simulink model "AMCLIB_FW_BAM_F32"  (Simulink 8.3)
settings: Solver=ode45  StartTime=0.0  StopTime=10.0  RelTol=1e-3
undefined symbols (not defined in the file): f32IntegGainFW, f32PropGainFW, s16IntegGainShiftFW, s16PropGainShiftFW, u16NSamplesFW
settings Model: Creator=B37097  LastModifiedBy=B37097
settings DataIOCC: SignalLoggingSaveFormat=Dataset
settings DebuggingCC: UnderspecifiedInitializationDetection=Simplified  StateNameClashWarn=none
settings GRTTargetCC: CombineOutputUpdateFcns=on  GRTInterface=off

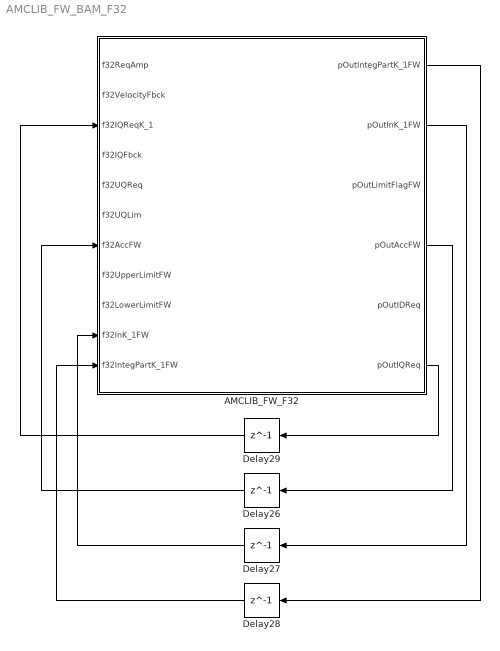
== system AMCLIB_FW_BAM_F32 ==
  AMCLIB_FW_F32 : Subsystem  mask(AMCLIB_FW_F32){u16NSamplesFW=u16NSamplesFW, f32PropGainFW=f32PropGainFW, s16PropGainShiftFW=s16PropGainShiftFW, f32IntegGainFW=f32IntegGainFW, s16IntegGainShiftFW=s16IntegGainShiftFW}
      mask help: Bit accurate model of the speed loop algorithm with field weakening capability in 32-bit fixed-point implementation.
      mask init:
      | pos = get_param(gcb, 'Position');width = pos(3) - pos(1); height = pos(4) - pos(2);tX=width/2;tY=height*0.9;
      mask Display: color('black');port_label('input',1,'f32ReqAmp');port_label('input',2,'f32VelocityFbck');port_label('input',3,'f32IQReqK_1');port_label('input',4,'f32IQFbck');port_label('input',5,'f32UQReq');port_label('input',6,'f32UQLim');port_label('input',7,'f32AccFW');port_label('input',8,'f32UpperLimitFW');port_label('input',9,'f32LowerLimitFW');port_label('input',10,'f32InK_1FW');port_label('input',11,'f32IntegPartK_1FW');port_label('output',1,'pOutIntegPartK_1FW');port_label('output',2,'pOutInK_1FW');port_label('output',3,'pOutLimitFlagFW');port_label('output',4,'pOutAccFW');port_label('output',5,'pOutIDReq');port_label('output',6,'pOutIQReq');color('black');disp('AMCLIB_FW_F32');color('blue');text(tX,tY, 'BAM', 'horizontalAlignment', 'center');
  Delay{26..29} (4 alike) : Delay  DelayLength=1  InitialCondition=0
  wires:
  AMCLIB_FW_F32/6(pOutIQReq) -> Delay29/1
  Delay29/1 -> AMCLIB_FW_F32/3(f32IQReqK_1)
  AMCLIB_FW_F32/4(pOutAccFW) -> Delay26/1
  Delay26/1 -> AMCLIB_FW_F32/7(f32AccFW)
  AMCLIB_FW_F32/2(pOutInK_1FW) -> Delay27/1
  Delay27/1 -> AMCLIB_FW_F32/10(f32InK_1FW)
  AMCLIB_FW_F32/1(pOutIntegPartK_1FW) -> Delay28/1
  Delay28/1 -> AMCLIB_FW_F32/11(f32IntegPartK_1FW)

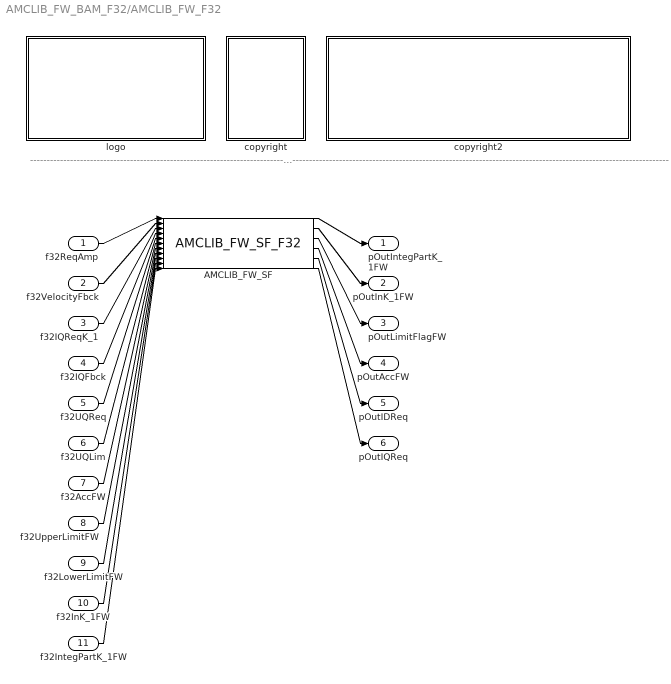
== system AMCLIB_FW_BAM_F32/AMCLIB_FW_F32 ==
  note: ---------------------------------------------------------------------------------------------------------------------------------------------------------------------------------------------------
  f32ReqAmp : Inport
  f32VelocityFbck : Inport  Port=2
  f32IQReqK_1 : Inport  Port=3
  f32IQFbck : Inport  Port=4
  f32UQReq : Inport  Port=5
  f32UQLim : Inport  Port=6
  f32AccFW : Inport  Port=7
  f32UpperLimitFW : Inport  Port=8
  f32LowerLimitFW : Inport  Port=9
  f32InK_1FW : Inport  Port=10
  f32IntegPartK_1FW : Inport  Port=11
  AMCLIB_FW_SF : S-Function  FunctionName=AMCLIB_FW_SF_F32  Parameters=u16NSamplesFW,f32PropGainFW,s16PropGainShiftFW,f32IntegGainFW,s16IntegGainShiftFW  EnableBusSupport=off
  copyright : Subsystem
      mask Display: text(10,90,'FILE:');text(10,75,'DESRIPTION:');text(10,60,'COPYRIGHT:');text(10,45,'VERSION:');text(10,30,'DATE:')
  copyright2 : Subsystem
      mask Display: text(10,90,'AMCLIB_FW_BAM_F32.mdl');text(10,75,'Speed Loop with Field Weakening.');text(10,60,'NXP');text(10,45,'1.0');text(10,30,'28-Aug-2017');
  logo : Subsystem
      mask Display: image(imread('logo.jpg'))
  pOutIntegPartK_1FW : Outport
  pOutInK_1FW : Outport  Port=2
  pOutLimitFlagFW : Outport  Port=3
  pOutAccFW : Outport  Port=4
  pOutIDReq : Outport  Port=5
  pOutIQReq : Outport  Port=6
  wires:
  f32ReqAmp/1 -> AMCLIB_FW_SF/1
  f32VelocityFbck/1 -> AMCLIB_FW_SF/2
  f32IQReqK_1/1 -> AMCLIB_FW_SF/3
  f32IQFbck/1 -> AMCLIB_FW_SF/4
  f32UQReq/1 -> AMCLIB_FW_SF/5
  f32UQLim/1 -> AMCLIB_FW_SF/6
  f32AccFW/1 -> AMCLIB_FW_SF/7
  f32UpperLimitFW/1 -> AMCLIB_FW_SF/8
  f32LowerLimitFW/1 -> AMCLIB_FW_SF/9
  f32InK_1FW/1 -> AMCLIB_FW_SF/10
  f32IntegPartK_1FW/1 -> AMCLIB_FW_SF/11
  AMCLIB_FW_SF/1 -> pOutIntegPartK_1FW/1
  AMCLIB_FW_SF/2 -> pOutInK_1FW/1
  AMCLIB_FW_SF/3 -> pOutLimitFlagFW/1
  AMCLIB_FW_SF/4 -> pOutAccFW/1
  AMCLIB_FW_SF/5 -> pOutIDReq/1
  AMCLIB_FW_SF/6 -> pOutIQReq/1

== system AMCLIB_FW_BAM_F32/AMCLIB_FW_F32/copyright ==

== system AMCLIB_FW_BAM_F32/AMCLIB_FW_F32/copyright2 ==

== system AMCLIB_FW_BAM_F32/AMCLIB_FW_F32/logo ==
